simulink library "motohawk_engine_motoshare_lib"  (Simulink 6.3)
undefined symbols (not defined in the file or in its folder): cast_val, IndPowerMax, lookup_group, motohawk_tex, motohawk_vardec_config_group, motohawk_vardec_path, SampleTime, SteadyStateECT, txtTitle, WarmUpTimeConst
libraries: MotoHawk_lib x211, motohawk_control_primitives_lib x20, motohawk_annotations_lib x7, motohawk_engine_lib x5, AutoDoc_lib x4, motohawk_control_primitives_lib_new x3, motohawk_control_primitives_motoshare_lib x2
(part 4 of 7)

== system motohawk_engine_motoshare_lib/Normalized Effective Combustion Chamber Temperature ==
  note: Only integrate while NECCT
      | is less than calibrated SteadyStateECT.
  IndPower [kW] : Inport
  ECT [degC] : Inport  Port=2
  CompareTo : Subsystem  mask(Equals){op===, val=0}
      mask prompts: op "Operator:"; val "Compare To:"
      mask help:
      | Check how input compares to 'n'.
      | Select an operation for comparison.
      | Any data type may be used for the value.  Real data type is based on input signal.
      mask init:
      | lbl = sprintf('in %s %d', op, double(val));
      | set_param([gcb '/RelOp'], 'Operator', op);
      mask StyleString: popup(==|~=|<|<=|>|>=),edit
      mask Display:
      | patch([0 0 1 1], 1.2*[0 0.075 0.075 0], [230/255 0/255 0/255])
      | patch([0 0 1 1], 1.2*[0.025 0.05 0.05 0.025], [150/255 0/255 0/255])
      | patch([0 0 1 1], 1.2*[0 0.025 0.025 0], [0/255 0/255 0/255])
      | 
      | disp(lbl);
  Integrate an offset to ECT  Reset offset when engine is stopped. : Subsystem
  Product : Product  Inputs=*/  SaturateOnIntegerOverflow=on  InputSameDT=on
  Product1 : Product  Inputs=***/  SaturateOnIntegerOverflow=on  InputSameDT=on
  Relational Operator : RelationalOperator  Operator=<  InputSameDT=on
  Sum : Sum  Inputs=+-|  SaturateOnIntegerOverflow=on  InputSameDT=on
  Sum1 : Sum  Inputs=++|  SaturateOnIntegerOverflow=on  InputSameDT=on
  Unit Delay : UnitDelay  Orientation=left  SampleTime=-1
  motohawk_TitleBlock : Subsystem  mask{BlockType_='Mototron_Title_Block', ttl='Normalized Effective Combustion Chamber Temperature (NECCT)\newline\rmUse engine power to model the temperature in the cylinder,\newlinenormalized to approach steady-state ECT over time.\newlineInstead of using ECT, which warms up more slowly than the cylinder itself, \newlineNECCT is used as the ordinate for warm-up tables.', im=mh.jpg}
      mask prompts: ttl "Description"; im "Image FIle"
      mask init:
      | set_param(gcb,'BlockType_','''Mototron_Title_Block''')
      | set_param(gcb,'MaskVisibilityString','off,on,on');
      mask Display:
      | image(imread(im),[0.31 0.66 0.31 0.35])
      | 
      | plot([0 0 1 1 0],[0 1 1 0 0])
      | plot([.3 1],[0.65 0.65])
      | plot([.3 .3],[0.1 1.0])
      | plot([0 1],[0.1 0.1])
      | plot([0.91 0.91],[0 0.1])
      | text(1,1,'\fontsize{22}\it\fontname{Arial Black}MotoTron Corporation \fontname{Arial}\fontsize{10}\newline505 Marion Road, Oshkosh, WI, 54901\newlinewww.mototron.com (734) 822-7700','verticalAlignment','Top','horizontalAlignment','Right','texmode','on')
      | text(0.01,1,['\fontsize{14}\it\bfPROPRIETARY\newlineAND CONFIDENTIAL\newline\fontsize{10}
      | THE INFORMATION CONTAINED IN THIS\newline
      | DRAWING IS THE SOLE PROPERTY OF\newline
      | MOTOTRON.  ANY REPRODUCTION IN\newline
      | PART OR AS A WHOLE WITHOUT THE\newline
      | WRITTEN PERMISSION OF MOTOTRON\newline
      | IS PROHIBITED.\fontsize{16}\rm\copyright\rm\fontsize{10} 2004' ],'verticalAlignment','Top','horizontalAlignment','Left','texmode','on')
      | 
      | text(0.9,0,['\fontsize{11}\bfPath: \rm' strrep(motohawk_vardec_path(gcb),'_','\_')],'verticalAlignment','Bottom','horizontalAlignment','Right','texmode','on')
      | text(0.31,0.65,['\fontsize{10}\bfDescription:'],'verticalAlignment','Top','horizontalAlignment','Left','texmode','on')
      | 
      | text(0.31,0.55,['\fontsize{14}\bf' ttl],'verticalAlignment','Top','horizontalAlignment','Left','texmode','on')
      | text(0.99,0,['\fontsize{11}\bfREV: \rm' motohawk_build_version],'verticalAlignment','Bottom','horizontalAlignment','Right','texmode','on')
  motohawk_calibration : S-Function  FunctionName=motohawk_sfun_calibration  Parameters=char({nam,''}), cast_val, uint8(storage), char({mototune_group,''}), min_val, max_val, char({help,''}), char({units,''}), boolean(inherit_dt), char({precision,''}), gain, offset, exp, read_level, write_level, uint8(view_as), char({enum_str,''})  mask(MotoHawk Calibration){nam='IndPowerMax', val=IndPowerMax, storage=Calibration, show_more=on, name_source=Use Parameter, data_type=Inherit from 'Default Value', read_level=1, write_level=1, view_as=Number, enum_struct={'Disabled', 'Enabled'}, use_help_units=on, help='Maximum indicated engine power', units='kW', use_min_max=on, min_val=0, max_val=1000, use_precision=off, precision='', gain=1, offset=0, exp=1, use_mototune_group=on, mototune_group=lookup_group(gcb)}
      mask prompts: nam "Name"; val "Default Value"; storage "Behavior"; show_more "------------ Show Additional Parameters ------------"; name_source "Name Source"; data_type "Output Data Type"; read_level "Read Access Level"; write_level "Write Access Level"; view_as "View Value As"; enum_struct "Enumeration (Cell String, or Struct)"; use_help_units "------ Show MotoTune Help and Units ------"; help "Help Text"; use_min_max "------ Show Min and Max Values ------"; min_val "Minimum Value"; max_val "Maximum Value"; use_precision "------ Show MotoTune Precision, Gain/Offset/Exponent ------"; exp "Exponent"; use_mototune_group "------ Show MotoTune Group ------"; mototune_group "MotoTune Group String"
      mask help:
      | This block provides a connection to MotoTune, and allows run-time modification of calibration values with the MotoTune tool.
      |
      | The block behaves in simulation like a Constant block, and accepts any Matlab value as its Default Value, including data-typing casts.
      |
      | Engineering Value = (Raw Module Value*Gain)^Exp)+Offset
      |
      | Press Help for more information.
      |
      | ---------------------------------------------------------------------
      | Copyright 2004 MotoTron, Inc.  All Rights Reserved.
      mask init:
      | dp = get_param(gcb, 'DialogParameters');
      | 
      | if (name_source == 2)
      | 	phs = get_param(gcb, 'PortHandles');
      | 	line = get_param(phs.Outport, 'Line');
      | 	if (line >= 0)
      | 		nam = get_param(line, 'Name');
      | 		nam = regexprep(nam, '[<>]', '');
      | 	else
      | 		nam = '';
      | 	end
      | end
      | 
      | lbl_name = nam;
      | if (length(lbl_name) == 0)
      | 	lbl_name = '(Undefined Name)';
      | end
      | 
      | if ischar(val)
      | 	val = uint8(val);
      | end
      | 
      | % Convert to selected data type
      | inherit_dt = false;
      | switch (data_type)
      | 	case 1, cast_val = val;
      | 	case 2, cast_val = double(val);  inherit_dt = true;
      | 	case 3, cast_val = double(val);
      | 	case 4, cast_val = single(val);
      | 	case 5, cast_val = int8(val);
      | 	case 6, cast_val = uint8(val);
      | 	case 7, cast_val = int16(val);
      | 	case 8, cast_val = uint16(val);
      | 	case 9, cast_val = int32(val);
      | 	case 10, cast_val = uint32(val);
      | 	case 11, cast_val = boolean(val);
      | end
      | 
      | if (view_as == 3)
      | 	lbl_val = sprintf('"%s"', char(val));
      | else
      | 	disp_val = ((double(cast_val) .* double(gain)) .^ double(exp)) + double(offset);
      | 	lbl_val = mat2str(disp_val, 5);
      | end
      | lbl_storage = dp.storage.Enum{storage};
      | lbl = [lbl_name  ' = '  lbl_val '\n(' lbl_storage ')'];
      | 
      | if (use_min_max & (max_val < min_val))
      | 	warning([gcb ': Maximum value must be greater than the minimum value']);
      | end
      | 
      | enum_str = '';
      | if (view_as == 2)
      | 	enum_str = motohawk_enum_to_string(enum_struct);
      | end
      mask Help:
      | <h3>Name:</h3>
      | When specifying a name, it  is treated as an evaluation string.
      | 
      | <h3>Default Value:</h3>
      | This is the value that is loaded before calibration through MotoTune.  This block will behave as a constant block that will output the Default Value.
      | 
      | <h3>Storage Classes:</h3>
      | <ul>
      | <li>Display - Default is reloaded on every power-up.  Volatile copy is tunable from the Display page.</li>
      | <li>Calibration - Default value is loaded when programmed.  Persistent value is tunable from the Calibration page.  Values may be uploaded & downloaded via a .cal file.</li>
      | </ul>
      | 
      | <h3>View as Enumeration</h3>
      | When checked, the Enumeration parameter is used to assign names to values, so that the names are visible in MotoTune, instead of the raw numeric values.
      | The Enumeration parameter may be defined in two ways:
      | <ul>
      | <li>Cell String:  A cell array of strings such as <i>{'Off', 'On'}</i> may be used to define the names of enumerated values.  In this case, the values start with 0 and increment by one.  This is especially useful for defining names for boolean flags like 'On' and 'Off'.
      | <li>Struct:  A Matlab struct array containing a 'name' field, and optionally a 'value' field may be used to define the names and explicitly define the values of an enumerated type.  For example:  <i>struct('name', {'Off', 'On'}, 'value', {0,1})</i>.  If the 'value' field is missing, then the values start with 0 and increment by one, just like with the Cell String format.
      | </ul>
      | Note that only integer or boolean values may be used with enumerations.  Floating point types such as double and single are not allowed.
      | 
      | <h3>Name Sources:</h3>
      | <ul>
      | <li>Use Parameter - The value is entered in the name field.   Note that this field is an expression, so literal strings must be surrounded by single quotes.</li>
      | <li>Use Output Wire Name - The name follows from the output wire name.</li>
      | </ul>
      | If no name is given, or if the name is invalid, (Undefined Name) will be displayed on the block.<\li>
      | 
      | <h3>Output Data Type:</h3>
      | Explicitly specify a data type, inherit the data type from the Default Value, or back propagate the data type from the attached Simulink signals.
      | 
      | <h3>Specify MotoTune Help and Units:</h3>
      | This is the help text and units that are displayed in MotoTune when calibrating this value.  Use this to provide information to the MotoTune user.
      | 
      | <h3>Specify Min and Max Values</h3>
      | The Minimum and maximum values are used by MotoTune to limit the the new calibrated value entered by the user inside of MotoTune.  This can be used to prevent a user from entering an out of bounds number when calibrating.
      | 
      | <h3>MotoTune Group String:</h3>
      | This is used to organize calibration and probe variables inside of MotoTune.  When a value is assigned to a group, it will appear under this group name as opposed to the default subsystem name.
      mask StyleString: edit,edit,popup(Startup Calibration|Calibration|Display),checkbox,popup(Use Parameter|Use Output Wire Name),popup(Inherit from 'Default Value'|Inherit via back propagation|double|single|int8|uint8|int16|uint16|int32|uint32|boolean),popup(1|2|3|4),popup(1|2|3|4),popup(Number|Enumeration|Text),edit,checkbox,edit,edit,checkbox,edit,edit,checkbox,edit,edit,edit,edit,checkbox,edit
      mask CallbackString:
      | |||motohawk_calibration_visible(gcb, 'show_more');
      | |motohawk_param_visible(gcb, 'nam', strcmp(get_param(gcb, 'name_source'), 'Use Parameter'));
      | ||||motohawk_param_enable(gcb, 'enum_struct', strcmp(get_param(gcb, 'view_as'), 'Enumeration'));
      | ||motohawk_calibration_visible(gcb, 'use_help_units');|||motohawk_calibration_visible(gcb, 'use_min_max');
      | |||motohawk_calibration_visible(gcb, 'use_precision');|||||motohawk_calibration_visible(gcb, 'use_mototune_group');|
      mask Display:
      | patch([0 0 1 1], [0 1 1 0], [220/255 220/255 220/255])
      | patch([0 0 1 1], [0 0.075 0.075 0], [230/255 0/255 0/255])
      | patch([0 0 1 1], [0.025 0.05 0.05 0.025], [150/255 0/255 0/255])
      | patch([0 0 1 1], [0 0.025 0.025 0], [0/255 0/255 0/255])
      | 
      | disp(lbl);
  motohawk_calibration1 : S-Function  FunctionName=motohawk_sfun_calibration  Parameters=char({nam,''}), cast_val, uint8(storage), char({mototune_group,''}), min_val, max_val, char({help,''}), char({units,''}), boolean(inherit_dt), char({precision,''}), gain, offset, exp, read_level, write_level, uint8(view_as), char({enum_str,''})  mask(MotoHawk Calibration){nam='SteadyStateECT', val=SteadyStateECT, storage=Calibration, show_more=on, name_source=Use Parameter, data_type=Inherit from 'Default Value', read_level=1, write_level=1, view_as=Number, enum_struct={'Disabled', 'Enabled'}, use_help_units=on, help='Steady state engine coolant temperature', units='degC', use_min_max=on, min_val=0, max_val=200, use_precision=off, precision='', gain=1, offset=0, exp=1, use_mototune_group=on, mototune_group=lookup_group(gcb)}
      mask prompts: nam "Name"; val "Default Value"; storage "Behavior"; show_more "------------ Show Additional Parameters ------------"; name_source "Name Source"; data_type "Output Data Type"; read_level "Read Access Level"; write_level "Write Access Level"; view_as "View Value As"; enum_struct "Enumeration (Cell String, or Struct)"; use_help_units "------ Show MotoTune Help and Units ------"; help "Help Text"; use_min_max "------ Show Min and Max Values ------"; min_val "Minimum Value"; max_val "Maximum Value"; use_precision "------ Show MotoTune Precision, Gain/Offset/Exponent ------"; exp "Exponent"; use_mototune_group "------ Show MotoTune Group ------"; mototune_group "MotoTune Group String"
      mask help:
      | This block provides a connection to MotoTune, and allows run-time modification of calibration values with the MotoTune tool.
      |
      | The block behaves in simulation like a Constant block, and accepts any Matlab value as its Default Value, including data-typing casts.
      |
      | Engineering Value = (Raw Module Value*Gain)^Exp)+Offset
      |
      | Press Help for more information.
      |
      | ---------------------------------------------------------------------
      | Copyright 2004 MotoTron, Inc.  All Rights Reserved.
      mask init: same as motohawk_engine_motoshare_lib/Normalized Effective Combustion Chamber Temperature/motohawk_calibration
      mask Help:
      | <h3>Name:</h3>
      | When specifying a name, it  is treated as an evaluation string.
      | 
      | <h3>Default Value:</h3>
      | This is the value that is loaded before calibration through MotoTune.  This block will behave as a constant block that will output the Default Value.
      | 
      | <h3>Storage Classes:</h3>
      | <ul>
      | <li>Display - Default is reloaded on every power-up.  Volatile copy is tunable from the Display page.</li>
      | <li>Calibration - Default value is loaded when programmed.  Persistent value is tunable from the Calibration page.  Values may be uploaded & downloaded via a .cal file.</li>
      | </ul>
      | 
      | <h3>View as Enumeration</h3>
      | When checked, the Enumeration parameter is used to assign names to values, so that the names are visible in MotoTune, instead of the raw numeric values.
      | The Enumeration parameter may be defined in two ways:
      | <ul>
      | <li>Cell String:  A cell array of strings such as <i>{'Off', 'On'}</i> may be used to define the names of enumerated values.  In this case, the values start with 0 and increment by one.  This is especially useful for defining names for boolean flags like 'On' and 'Off'.
      | <li>Struct:  A Matlab struct array containing a 'name' field, and optionally a 'value' field may be used to define the names and explicitly define the values of an enumerated type.  For example:  <i>struct('name', {'Off', 'On'}, 'value', {0,1})</i>.  If the 'value' field is missing, then the values start with 0 and increment by one, just like with the Cell String format.
      | </ul>
      | Note that only integer or boolean values may be used with enumerations.  Floating point types such as double and single are not allowed.
      | 
      | <h3>Name Sources:</h3>
      | <ul>
      | <li>Use Parameter - The value is entered in the name field.   Note that this field is an expression, so literal strings must be surrounded by single quotes.</li>
      | <li>Use Output Wire Name - The name follows from the output wire name.</li>
      | </ul>
      | If no name is given, or if the name is invalid, (Undefined Name) will be displayed on the block.<\li>
      | 
      | <h3>Output Data Type:</h3>
      | Explicitly specify a data type, inherit the data type from the Default Value, or back propagate the data type from the attached Simulink signals.
      | 
      | <h3>Specify MotoTune Help and Units:</h3>
      | This is the help text and units that are displayed in MotoTune when calibrating this value.  Use this to provide information to the MotoTune user.
      | 
      | <h3>Specify Min and Max Values</h3>
      | The Minimum and maximum values are used by MotoTune to limit the the new calibrated value entered by the user inside of MotoTune.  This can be used to prevent a user from entering an out of bounds number when calibrating.
      | 
      | <h3>MotoTune Group String:</h3>
      | This is used to organize calibration and probe variables inside of MotoTune.  When a value is assigned to a group, it will appear under this group name as opposed to the default subsystem name.
      mask StyleString: edit,edit,popup(Startup Calibration|Calibration|Display),checkbox,popup(Use Parameter|Use Output Wire Name),popup(Inherit from 'Default Value'|Inherit via back propagation|double|single|int8|uint8|int16|uint16|int32|uint32|boolean),popup(1|2|3|4),popup(1|2|3|4),popup(Number|Enumeration|Text),edit,checkbox,edit,edit,checkbox,edit,edit,checkbox,edit,edit,edit,edit,checkbox,edit
      mask CallbackString:
      | |||motohawk_calibration_visible(gcb, 'show_more');
      | |motohawk_param_visible(gcb, 'nam', strcmp(get_param(gcb, 'name_source'), 'Use Parameter'));
      | ||||motohawk_param_enable(gcb, 'enum_struct', strcmp(get_param(gcb, 'view_as'), 'Enumeration'));
      | ||motohawk_calibration_visible(gcb, 'use_help_units');|||motohawk_calibration_visible(gcb, 'use_min_max');
      | |||motohawk_calibration_visible(gcb, 'use_precision');|||||motohawk_calibration_visible(gcb, 'use_mototune_group');|
      mask Display:
      | patch([0 0 1 1], [0 1 1 0], [220/255 220/255 220/255])
      | patch([0 0 1 1], [0 0.075 0.075 0], [230/255 0/255 0/255])
      | patch([0 0 1 1], [0.025 0.05 0.05 0.025], [150/255 0/255 0/255])
      | patch([0 0 1 1], [0 0.025 0.025 0], [0/255 0/255 0/255])
      | 
      | disp(lbl);
  motohawk_calibration2 : S-Function  FunctionName=motohawk_sfun_calibration  Parameters=char({nam,''}), cast_val, uint8(storage), char({mototune_group,''}), min_val, max_val, char({help,''}), char({units,''}), boolean(inherit_dt), char({precision,''}), gain, offset, exp, read_level, write_level, uint8(view_as), char({enum_str,''})  mask(MotoHawk Calibration){nam='WarmUpTimeConst', val=WarmUpTimeConst, storage=Calibration, show_more=on, name_source=Use Parameter, data_type=Inherit from 'Default Value', read_level=1, write_level=1, view_as=Number, enum_struct={'Disabled', 'Enabled'}, use_help_units=on, help='Warm-up time constant.  Determines how quickly NECCT warms up relative to ECT.', units='sec', use_min_max=on, min_val=SampleTime, max_val=10000, use_precision=off, precision='', gain=1, offset=0, exp=1, use_mototune_group=on, mototune_group=lookup_group(gcb)}
      mask prompts: nam "Name"; val "Default Value"; storage "Behavior"; show_more "------------ Show Additional Parameters ------------"; name_source "Name Source"; data_type "Output Data Type"; read_level "Read Access Level"; write_level "Write Access Level"; view_as "View Value As"; enum_struct "Enumeration (Cell String, or Struct)"; use_help_units "------ Show MotoTune Help and Units ------"; help "Help Text"; use_min_max "------ Show Min and Max Values ------"; min_val "Minimum Value"; max_val "Maximum Value"; use_precision "------ Show MotoTune Precision, Gain/Offset/Exponent ------"; exp "Exponent"; use_mototune_group "------ Show MotoTune Group ------"; mototune_group "MotoTune Group String"
      mask help:
      | This block provides a connection to MotoTune, and allows run-time modification of calibration values with the MotoTune tool.
      |
      | The block behaves in simulation like a Constant block, and accepts any Matlab value as its Default Value, including data-typing casts.
      |
      | Engineering Value = (Raw Module Value*Gain)^Exp)+Offset
      |
      | Press Help for more information.
      |
      | ---------------------------------------------------------------------
      | Copyright 2004 MotoTron, Inc.  All Rights Reserved.
      mask init: same as motohawk_engine_motoshare_lib/Normalized Effective Combustion Chamber Temperature/motohawk_calibration
      mask Help:
      | <h3>Name:</h3>
      | When specifying a name, it  is treated as an evaluation string.
      | 
      | <h3>Default Value:</h3>
      | This is the value that is loaded before calibration through MotoTune.  This block will behave as a constant block that will output the Default Value.
      | 
      | <h3>Storage Classes:</h3>
      | <ul>
      | <li>Display - Default is reloaded on every power-up.  Volatile copy is tunable from the Display page.</li>
      | <li>Calibration - Default value is loaded when programmed.  Persistent value is tunable from the Calibration page.  Values may be uploaded & downloaded via a .cal file.</li>
      | </ul>
      | 
      | <h3>View as Enumeration</h3>
      | When checked, the Enumeration parameter is used to assign names to values, so that the names are visible in MotoTune, instead of the raw numeric values.
      | The Enumeration parameter may be defined in two ways:
      | <ul>
      | <li>Cell String:  A cell array of strings such as <i>{'Off', 'On'}</i> may be used to define the names of enumerated values.  In this case, the values start with 0 and increment by one.  This is especially useful for defining names for boolean flags like 'On' and 'Off'.
      | <li>Struct:  A Matlab struct array containing a 'name' field, and optionally a 'value' field may be used to define the names and explicitly define the values of an enumerated type.  For example:  <i>struct('name', {'Off', 'On'}, 'value', {0,1})</i>.  If the 'value' field is missing, then the values start with 0 and increment by one, just like with the Cell String format.
      | </ul>
      | Note that only integer or boolean values may be used with enumerations.  Floating point types such as double and single are not allowed.
      | 
      | <h3>Name Sources:</h3>
      | <ul>
      | <li>Use Parameter - The value is entered in the name field.   Note that this field is an expression, so literal strings must be surrounded by single quotes.</li>
      | <li>Use Output Wire Name - The name follows from the output wire name.</li>
      | </ul>
      | If no name is given, or if the name is invalid, (Undefined Name) will be displayed on the block.<\li>
      | 
      | <h3>Output Data Type:</h3>
      | Explicitly specify a data type, inherit the data type from the Default Value, or back propagate the data type from the attached Simulink signals.
      | 
      | <h3>Specify MotoTune Help and Units:</h3>
      | This is the help text and units that are displayed in MotoTune when calibrating this value.  Use this to provide information to the MotoTune user.
      | 
      | <h3>Specify Min and Max Values</h3>
      | The Minimum and maximum values are used by MotoTune to limit the the new calibrated value entered by the user inside of MotoTune.  This can be used to prevent a user from entering an out of bounds number when calibrating.
      | 
      | <h3>MotoTune Group String:</h3>
      | This is used to organize calibration and probe variables inside of MotoTune.  When a value is assigned to a group, it will appear under this group name as opposed to the default subsystem name.
      mask StyleString: edit,edit,popup(Startup Calibration|Calibration|Display),checkbox,popup(Use Parameter|Use Output Wire Name),popup(Inherit from 'Default Value'|Inherit via back propagation|double|single|int8|uint8|int16|uint16|int32|uint32|boolean),popup(1|2|3|4),popup(1|2|3|4),popup(Number|Enumeration|Text),edit,checkbox,edit,edit,checkbox,edit,edit,checkbox,edit,edit,edit,edit,checkbox,edit
      mask CallbackString:
      | |||motohawk_calibration_visible(gcb, 'show_more');
      | |motohawk_param_visible(gcb, 'nam', strcmp(get_param(gcb, 'name_source'), 'Use Parameter'));
      | ||||motohawk_param_enable(gcb, 'enum_struct', strcmp(get_param(gcb, 'view_as'), 'Enumeration'));
      | ||motohawk_calibration_visible(gcb, 'use_help_units');|||motohawk_calibration_visible(gcb, 'use_min_max');
      | |||motohawk_calibration_visible(gcb, 'use_precision');|||||motohawk_calibration_visible(gcb, 'use_mototune_group');|
      mask Display:
      | patch([0 0 1 1], [0 1 1 0], [220/255 220/255 220/255])
      | patch([0 0 1 1], [0 0.075 0.075 0], [230/255 0/255 0/255])
      | patch([0 0 1 1], [0.025 0.05 0.05 0.025], [150/255 0/255 0/255])
      | patch([0 0 1 1], [0 0.025 0.025 0], [0/255 0/255 0/255])
      | 
      | disp(lbl);
  motohawk_delta_time : S-Function  FunctionName=motohawk_sfun_delta_time  Parameters=samp_time, double(init_val)  mask(MotoHawk Delta Time){samp_time=SampleTime, init_val=0}
      mask prompts: samp_time "Sample Time"; init_val "Initial Value"
      mask help:
      | Outputs the delta time since the last time this block was called (in seconds).
      |
      | If a positive 'Sample Time' is entered, this constant value will be output every time.  The output data type will be the same as the 'Sample Time' parameter.  In this case, the 'Initial Value' parameter is unused.
      |
      | If a zero or negative 'Sample Time' is entered, the block will calculate the delta time, and the block\ will output 'Initial Value' the first time it is called.
      |
      | Using a constant sample time is more efficient than an inherited sample time, because it does not generate extra code and RAM to dynamically calculate the delta time.
      |
      | Note that the block still runs with inherited sample-time in the Simulink environment, regardless of what is entered.  It is legal to insert a 'wrong' value into the Sample Time (a value that doesn't actually represent the number of seconds between executions), and the block will happily output that value.
      |
      | ---------------------------------------------------------------------
      | Copyright 2004 MotoTron, Inc.  All Rights Reserved.
      mask Display:
      | patch([0 0 1 1], [0 1 1 0], [220/255 220/255 220/255])
      | patch([0 0 1 1], [0 0.075 0.075 0], [230/255 0/255 0/255])
      | patch([0 0 1 1], [0.025 0.05 0.05 0.025], [150/255 0/255 0/255])
      | patch([0 0 1 1], [0 0.025 0.025 0], [0/255 0/255 0/255])
      | 
      | disp('dT');
  motohawk_probe : S-Function  FunctionName=motohawk_sfun_probe  Parameters=char({nam,''}), char({mototune_group,''}), char({help,''}), char({units,''}), char({precision,''}), gain, offset, exp, read_level, uint8(view_as), char({enum_str,''})  mask(MotoHawk Probe){nam='NECCT', show_more=on, name_source=Use Parameter, read_level=1, view_as=Number, enum_struct={'Disabled', 'Enabled'}, use_help_units=on, help='Normalized effective combustion chamber temperature', units='degC', use_precision=off, precision='', gain=1, offset=0, exp=1, use_mototune_group=on, mototune_group=lookup_group(gcb)}
      mask prompts: nam "Name"; show_more "------------ Show Additional Parameters ------------"; name_source "Name Source"; read_level "Read Access Level"; view_as "View Value As"; enum_struct "Enumeration (Cell String, or Struct)"; use_help_units "------ Show MotoTune Help and Units ------"; help "Help Text"; use_precision "------ Show MotoTune Precision, Gain/Offset/Exponent ------"; exp "Exponent"; use_mototune_group "------ Show MotoTune Group ------"; mototune_group "MotoTune Group String"
      mask help:
      | This block provides a connection to MotoTune, and allows run-time observation of probed values with the MotoTune tool.
      |
      | The Name Source field allows the name to be entered as a Literal, evaluated as a Matlab expression, or it may be inherited from the name of the input wire.  If no name is supplied, (Undefined Name) will be displayed on the block.
      |
      | Engineering Value = (Raw Module Value*Gain)^Exp)+Offset
      |
      | Press Help for more information.
      |
      | ---------------------------------------------------------------------
      | Copyright 2004 MotoTron, Inc.  All Rights Reserved.
      mask init:
      | if (name_source == 2)
      | 	phs = get_param(gcb, 'PortHandles');
      | 	line = get_param(phs.Inport, 'Line');
      | 	if (line >= 0)
      | 		nam = get_param(line, 'Name');
      | 		nam = regexprep(nam, '[<>]', '');
      | 	else
      | 		nam = '';
      | 	end
      | end
      | 
      | lbl_name = nam;
      | if (length(lbl_name) == 0)
      | 	lbl_name = '(Undefined Name)';
      | end
      | 
      | enum_str = '';
      | if (view_as == 2)
      | 	enum_str = motohawk_enum_to_string(enum_struct);
      | end
      mask Help:
      | <h3>Name:</h3>
      | When specifying a name, it  is treated as an evaluation string.
      | 
      | <h3>View as Enumeration</h3>
      | When checked, the Enumeration parameter is used to assign names to values, so that the names are visible in MotoTune, instead of the raw numeric values.
      | The Enumeration parameter may be defined in two ways:
      | <ul>
      | <li>Cell String:  A cell array of strings such as <i>{'Off', 'On'}</i> may be used to define the names of enumerated values.  In this case, the values start with 0 and increment by one.  This is especially useful for defining names for boolean flags like 'On' and 'Off'.
      | <li>Struct:  A Matlab struct array containing a 'name' field, and optionally a 'value' field may be used to define the names and explicitly define the values of an enumerated type.  For example:  <i>struct('name', {'Off', 'On'}, 'value', {0,1})</i>.  If the 'value' field is missing, then the values start with 0 and increment by one, just like with the Cell String format.
      | </ul>
      | Note that only integer or boolean values may be used with enumerations.  Floating point types such as double and single are not allowed.
      | 
      | <h3>Name Sources:</h3>
      | <ul>
      | <li>Use Parameter - The value is entered in the name field.   Note that this field is an expression, so literal strings must be surrounded by single quotes.</li>
      | <li>Use Input Wire Name - The name follows from the input wire name.</li>
      | </ul>
      | If no name is given, or if the name is invalid, (Undefined Name) will be displayed on the block.<\li>
      | 
      | <h3>Specify MotoTune Help and Units:</h3>
      | This is the help text and units that are displayed in MotoTune when probing this value.  Use this to provide information to the MotoTune user.
      | 
      | <h3>MotoTune Group String:</h3>
      | This is used to organize calibration and probe variables inside of MotoTune.  When a value is assigned to a group, it will appear under this group name as opposed to the default subsystem name.
      mask StyleString: edit,checkbox,popup(Use Parameter|Use Input Wire Name),popup(1|2|3|4),popup(Number|Enumeration|Text),edit,checkbox,edit,edit,checkbox,edit,edit,edit,edit,checkbox,edit
      mask CallbackString:
      | |motohawk_probe_visible(gcb, 'show_more');
      | |use = strmatch(get_param(gcb, 'name_source'), 'Use Parameter', 'exact');
      | motohawk_param_visible(gcb, 'nam', use);
      | ||motohawk_param_enable(gcb, 'enum_struct', strcmp(get_param(gcb, 'view_as'), 'Enumeration'));
      | ||motohawk_probe_visible(gcb, 'use_help_units');|||motohawk_probe_visible(gcb, 'use_precision');|||||motohawk_probe_visible(gcb, 'use_mototune_group');|
      mask Display:
      | patch([0 0 1 1], [0 1 1 0], [220/255 220/255 220/255])
      | patch([0 0 1 1], [0 0.075 0.075 0], [230/255 0/255 0/255])
      | patch([0 0 1 1], [0.025 0.05 0.05 0.025], [150/255 0/255 0/255])
      | patch([0 0 1 1], [0 0.025 0.025 0], [0/255 0/255 0/255])
      | 
      | disp(lbl_name);
  NECCT [degC] : Outport
  wires:
  IndPower [kW]/1 -> Product/1, CompareTo/1(In)
  motohawk_calibration/1 -> Product/2
  motohawk_calibration1/1 -> Sum/1, Relational Operator/2
  ECT [degC]/1 -> Sum/2, Sum1/1
  Sum/1 -> Product1/1
  Product/1 -> Product1/2
  motohawk_delta_time/1 -> Product1/3
  motohawk_calibration2/1 -> Product1/4
  Product1/1 -> Integrate an offset to ECT  Reset offset when engine is stopped./1(Integrand)
  CompareTo/1(Out) -> Integrate an offset to ECT  Reset offset when engine is stopped./2(Reset)
  Relational Operator/1 -> Integrate an offset to ECT  Reset offset when engine is stopped./Enable
  Unit Delay/1 -> Relational Operator/1
  Integrate an offset to ECT  Reset offset when engine is stopped./1(ECT Offset) -> Sum1/2
  Sum1/1 -> motohawk_probe/1, NECCT [degC]/1, Unit Delay/1

== system motohawk_engine_motoshare_lib/O2A ==
  O2Sensor : Inport
  DesEquivRatio : Inport  Port=2
  Enable : EnablePort
  Bus Selector : BusSelector  OutputSignals=RichEquivRatioTargetDelta,LeanEquivRatioTargetDelta,RichEquivRatioSwPtDelta,LeanEquivRatioSwPtDelta
  Bus Selector1 : BusSelector  OutputSignals=O2ControlErrorGain,O2ControlPGain,O2ControlIGain,O2ControlDGain,O2ControlITermUpperLimit,O2ControlItermLowerLimit,O2ControlOutUpperLimit,O2ControlOutLowerLimit
  Closed-Loop O2 PID Controller : Subsystem
  Equivalence Ratio Perturbation : Subsystem  Description=|
      | /* Name: PosPertMagnitude Unit:phi ClassID:VAR StorageID:FLASH Access:RW4+RW3+NA2+NA1 TypeID:UINT1               
      |    Gain:0.01 Min:0.00 Max:2.55 Format:5.2 UpdateID:REMOTE Group:"Engine Control | Run | Fuel | O2 Control | O2 " 
      |    "Control Config" Help:"Positive value added to EquivRatioWU for PosPertPeriod ms during the positive portion "
      |    "of the perturbation cycle. Used for catalyst efficiency optimization." VardecSig:6C */                       
      |                                                                                                                  
      | /* Name: NegPertMagnitude Unit:phi ClassID:VAR StorageID:FLASH Access:RW4+RW3+NA2+NA1 TypeID:UINT1               
      |    Gain:0.01 Min:0.00 Max:2.55 Format:5.2 UpdateID:REMOTE Group:"Engine Control | Run | Fuel | O2 Control | O2 " 
      |    "Control Config" Help:"Negative value added to EquivRatioWU for NegPertPeriod ms during the negative portion "
      |    "of the perturbation cycle. Used for catalyst efficiency optimization." VardecSig:6C */                       
      |                                                                                                                  
      | /* Name: PosPertPeriod Unit:ms ClassID:VAR StorageID:FLASH Access:RW4+RW3+NA2+NA1 TypeID:UINT1 Gain:5            
      |    Min:0.00 Max:1275.00 Format:5.2 UpdateID:REMOTE Group:"Engine Control | Run | Fuel | O2 Control | O2 "        
      |    "Control Config" Help:"Duration of the positive portion of the perturbation cycle. Used for catalyst "        
      |    "efficiency optimization." VardecSig:6C */                                                                    
      |                                                                                                                  
      | /* Name: NegPertPeriod Unit:ms ClassID:VAR StorageID:FLASH Access:RW4+RW3+NA2+NA1 TypeID:UINT1 Gain:5            
      |    Min:0.00 Max:1275.00 Format:5.2 UpdateID:REMOTE Group:"Engine Control | Run | Fuel | O2 Control | O2 "        
      |    "Control Config" Help:"Duration of the negative portion of the perturbation cycle. Used for catalyst "        
      |    "efficiency optimization." VardecSig:6C */
  Multiply by 1.0 if not yet enabled : InitialCondition  Value=1.0
  O2 Calibrations : Subsystem
  motohawk_TitleBlock : motohawk_annotations_lib/motohawk_TitleBlock  BlockType_='Mototron_Title_Block'  ttl=[txtTitle '\newline\rmClosed-Loop O2 for Bank ' bank]  copyright="'THE INFORMATION CONTAINED IN THIS\\newlineDRAWING IS THE SOLE PROPERTY OF\\newlineMOTOTRON.  ANY REPRODUCTION IN\\newline PART OR AS A WHOLE WITHOUT THE\\newlineWRITTEN PERMISSION OF MOTOTRON\\newline IS PROHIBITED.\\fontsize{16}\\rm\\copyright\\rm\\fontsize{10} 2005'"  address='\fontsize{22}\it\fontname{Arial Black}MotoTron Corporation \fontname{Arial}\fontsize{10}\newline505 Marion Road, Oshkosh, WI, 54901\newlinewww.mototron.com (734) 822-7700'  image_file='mh.jpg'  pretty_print=on  edit_text=[motohawk_tex(get_param(bdroot, 'Description')) '\rm\newline' motohawk_tex(get_param(gcs, 'Name'))]  edit_as=6
  motohawk_probe : MotoHawk_lib/Calibration & Probing Blocks/motohawk_probe  nam=['O2TargetEquivRatio' bank]  show_more=on  name_source=Use Parameter  read_level=1  view_as=Number  enum_struct={'Disabled', 'Enabled'}  vector_style=Wide Row  use_help_units=on  help=['Current target equivalence ratio for closed-loop O2 control, on bank ' bank]  units='ratio'  use_header_enum=off  row_header_enum={}  col_header_enum={}  use_precision=off  precision=''  gain=1  offset=0  exp=1  use_mototune_group=on  mototune_group=display_group
  FuelMult : Outport
  O2 Error : Outport  Port=2
  wires:
  Closed-Loop O2 PID Controller/2(ITerm) -> O2 Error/1
  Multiply by 1.0 if not yet enabled/1 -> FuelMult/1
  Bus Selector1/8 -> Closed-Loop O2 PID Controller/10(OutLowerLimit)  "<O2ControlOutLowerLimit>"
  Bus Selector1/7 -> Closed-Loop O2 PID Controller/9(OutUpperLimit)  "<O2ControlOutUpperLimit>"
  Bus Selector1/6 -> Closed-Loop O2 PID Controller/8(ITermLowerLimit)  "<O2ControlItermLowerLimit>"
  Bus Selector1/5 -> Closed-Loop O2 PID Controller/7(ITermUpperLimit)  "<O2ControlITermUpperLimit>"
  Bus Selector1/4 -> Closed-Loop O2 PID Controller/6(DGain)  "<O2ControlDGain>"
  Bus Selector1/3 -> Closed-Loop O2 PID Controller/5(IGain)  "<O2ControlIGain>"
  Bus Selector1/2 -> Closed-Loop O2 PID Controller/4(PGain)  "<O2ControlPGain>"
  Bus Selector1/1 -> Closed-Loop O2 PID Controller/3(ErrorGain)  "<O2ControlErrorGain>"
  Bus Selector/4 -> Equivalence Ratio Perturbation/6(LeanEquivRatioSwPtDelta)  "<LeanEquivRatioSwPtDelta>"
  Bus Selector/3 -> Equivalence Ratio Perturbation/5(RichEquivRatioSwPtDelta)  "<RichEquivRatioSwPtDelta>"
  Bus Selector/2 -> Equivalence Ratio Perturbation/4(LeanEquivRatioTargetDelta)  "<LeanEquivRatioTargetDelta>"
  Bus Selector/1 -> Equivalence Ratio Perturbation/3(RichEquivRatioTargetDelta)  "<RichEquivRatioTargetDelta>"
  O2 Calibrations/1(Calibrations) -> Bus Selector1/1, Bus Selector/1
  DesEquivRatio/1 -> Equivalence Ratio Perturbation/2(DesEquivRatio)
  Closed-Loop O2 PID Controller/1(Multiplier) -> Multiply by 1.0 if not yet enabled/1
  O2Sensor/1 -> Closed-Loop O2 PID Controller/1(O2Sensor), Equivalence Ratio Perturbation/1(O2Sensor)
  Equivalence Ratio Perturbation/1(Target Phi) -> motohawk_probe/1, Closed-Loop O2 PID Controller/2(TargetEquivRatio)

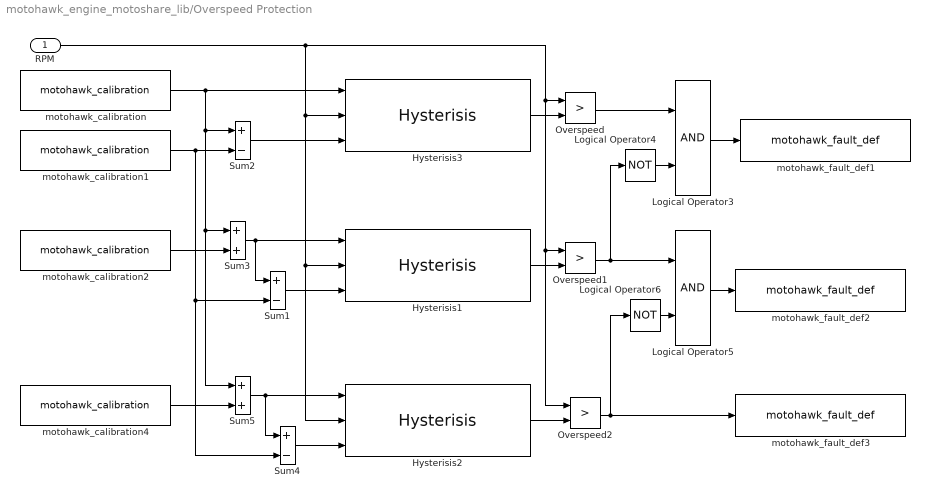
== system motohawk_engine_motoshare_lib/Overspeed Protection ==
  RPM : Inport
  Hysterisis1 : motohawk_control_primitives_lib_new/Hysterisis
  Hysterisis2 : motohawk_control_primitives_lib_new/Hysterisis
  Hysterisis3 : motohawk_control_primitives_lib_new/Hysterisis
  Logical Operator3 : Logic
  Logical Operator4 : Logic  Operator=NOT
  Logical Operator5 : Logic
  Logical Operator6 : Logic  Operator=NOT
  Overspeed : RelationalOperator  Operator=>  ZeroCross=off  InputSameDT=on
  Overspeed1 : RelationalOperator  Operator=>  ZeroCross=off  InputSameDT=on
  Overspeed2 : RelationalOperator  Operator=>  ZeroCross=off  InputSameDT=on
  Sum1 : Sum  Inputs=+-  SaturateOnIntegerOverflow=on
  Sum2 : Sum  Inputs=+-  SaturateOnIntegerOverflow=on
  Sum3 : Sum  SaturateOnIntegerOverflow=on
  Sum4 : Sum  Inputs=+-  SaturateOnIntegerOverflow=on
  Sum5 : Sum  SaturateOnIntegerOverflow=on
  motohawk_calibration : MotoHawk_lib/Calibration & Probing Blocks/motohawk_calibration  nam='BaseRevLimit'  val=2800  storage=Calibration  show_more=on  name_source=Use Parameter  data_type=Inherit from 'Default Value'  read_level=1  write_level=1  ovr_cals=on  view_as=Number  enum_struct={'Disabled', 'Enabled'}  vector_style=Wide Row  use_help_units=on  help='Maximum RPM allowed, before any action is taken'  units='RPM'  use_header_enum=off  row_header_enum={}  col_header_enum={}  use_min_max=on  min_val=0  max_val=inf  use_precision=off  precision=''  gain=1  offset=0  exp=1  use_mototune_group=on  mototune_group='Diagnostics & Protection | RevLimitConfig'
  motohawk_calibration1 : MotoHawk_lib/Calibration & Probing Blocks/motohawk_calibration  nam='RevLimitHyst'  val=20  storage=Calibration  show_more=on  name_source=Use Parameter  data_type=Inherit from 'Default Value'  read_level=1  write_level=1  ovr_cals=on  view_as=Number  enum_struct={'Disabled', 'Enabled'}  vector_style=Wide Row  use_help_units=on  help='Hysteresis applied to MaxRPM once rev limit threshold is satisfied'  units='RPM'  use_header_enum=off  row_header_enum={}  col_header_enum={}  use_min_max=on  min_val=0  max_val=12000  use_precision=off  precision=''  gain=1  offset=0  exp=1  use_mototune_group=on  mototune_group='Diagnostics & Protection | RevLimitConfig'
  motohawk_calibration2 : MotoHawk_lib/Calibration & Probing Blocks/motohawk_calibration  nam='MediumRevOffset'  val=75  storage=Calibration  show_more=on  name_source=Use Parameter  data_type=Inherit from 'Default Value'  read_level=1  write_level=1  ovr_cals=on  view_as=Number  enum_struct={'Disabled', 'Enabled'}  vector_style=Wide Row  use_help_units=on  help='RPM rev limit for medium action to be taken'  units='RPM'  use_header_enum=off  row_header_enum={}  col_header_enum={}  use_min_max=on  min_val=0  max_val=inf  use_precision=off  precision=''  gain=1  offset=0  exp=1  use_mototune_group=on  mototune_group='Diagnostics & Protection | RevLimitConfig'
  motohawk_calibration4 : MotoHawk_lib/Calibration & Probing Blocks/motohawk_calibration  nam='HardRevOffset'  val=100  storage=Calibration  show_more=on  name_source=Use Parameter  data_type=Inherit from 'Default Value'  read_level=1  write_level=1  ovr_cals=on  view_as=Number  enum_struct={'Disabled', 'Enabled'}  vector_style=Wide Row  use_help_units=on  help='RPM rev limit for hard action to be taken'  units='RPM'  use_header_enum=off  row_header_enum={}  col_header_enum={}  use_min_max=on  min_val=0  max_val=inf  use_precision=off  precision=''  gain=1  offset=0  exp=1  use_mototune_group=on  mototune_group='Diagnostics & Protection | RevLimitConfig'
  motohawk_fault_def1 : MotoHawk_lib/Fault Management Blocks/motohawk_fault_def  nam='SoftOverspeed'  mode=Enabled  id=[]  x=5  y=10  input_suspected=on  indeterminate=off  increment_xy=on  downsample_count=1  ovr_cals=on  ovr_actions=on  show_actions=off  action1_name=''  action1_cond=(None)  action2_name=''  action2_cond=(None)  action3_name=''  action3_cond=(None)  action4_name=''  action4_cond=(None)
  motohawk_fault_def2 : MotoHawk_lib/Fault Management Blocks/motohawk_fault_def  nam='MediumOverspeed'  mode=Enabled  id=[]  x=5  y=10  input_suspected=on  indeterminate=off  increment_xy=on  downsample_count=1  ovr_cals=on  ovr_actions=on  show_actions=off  action1_name=''  action1_cond=(None)  action2_name=''  action2_cond=(None)  action3_name=''  action3_cond=(None)  action4_name=''  action4_cond=(None)
  motohawk_fault_def3 : MotoHawk_lib/Fault Management Blocks/motohawk_fault_def  nam='HardOverspeed'  mode=Enabled  id=[]  x=5  y=10  input_suspected=on  indeterminate=off  increment_xy=on  downsample_count=1  ovr_cals=on  ovr_actions=on  show_actions=off  action1_name=''  action1_cond=(None)  action2_name=''  action2_cond=(None)  action3_name=''  action3_cond=(None)  action4_name=''  action4_cond=(None)
  wires:
  Hysterisis2/1 -> Overspeed2/2
  Hysterisis1/1 -> Overspeed1/2
  Hysterisis3/1 -> Overspeed/2
  motohawk_calibration1/1 -> Sum2/2, Sum1/2, Sum4/2
  motohawk_calibration/1 -> Sum2/1, Sum3/1, Sum5/1, Hysterisis3/1
  RPM/1 -> Overspeed/1, Overspeed1/1, Overspeed2/1, Hysterisis3/2, Hysterisis1/2, Hysterisis2/2
  motohawk_calibration2/1 -> Sum3/2
  Sum3/1 -> Sum1/1, Hysterisis1/1
  motohawk_calibration4/1 -> Sum5/2
  Sum5/1 -> Sum4/1, Hysterisis2/1
  Overspeed/1 -> Logical Operator3/1
  Logical Operator3/1 -> motohawk_fault_def1/1
  Logical Operator4/1 -> Logical Operator3/2
  Overspeed1/1 -> Logical Operator4/1, Logical Operator5/1
  Logical Operator6/1 -> Logical Operator5/2
  Overspeed2/1 -> Logical Operator6/1, motohawk_fault_def3/1
  Logical Operator5/1 -> motohawk_fault_def2/1
  Sum2/1 -> Hysterisis3/3
  Sum1/1 -> Hysterisis1/3
  Sum4/1 -> Hysterisis2/3
